simulink model "del3_linjefolging"  (R2024a)
settings: Solver=VariableStepAuto  StartTime=0.0  StopTime=inf  RelTol=1e-3
InitFcn:
  | id_setup()
StartFcn:
  | c_id = evalin('base', "car_id");
  | g_id = evalin('base', "group_id");
  | mqttBasic(c_id,g_id);
libraries: send x3, read x1, init x1
settings Model: Creator=eikel  LastModifiedBy=adriaeik

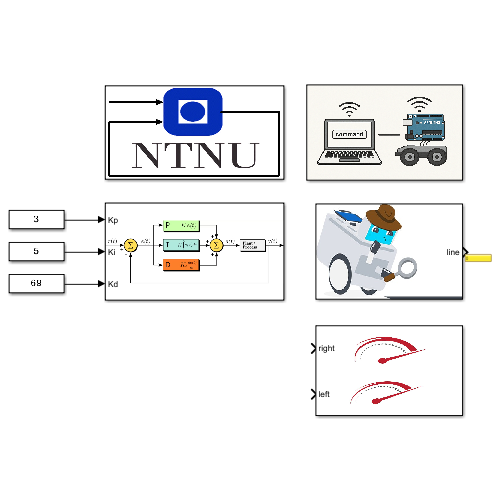
[thumbnail: Simulink's stored preview of the top-level diagram]
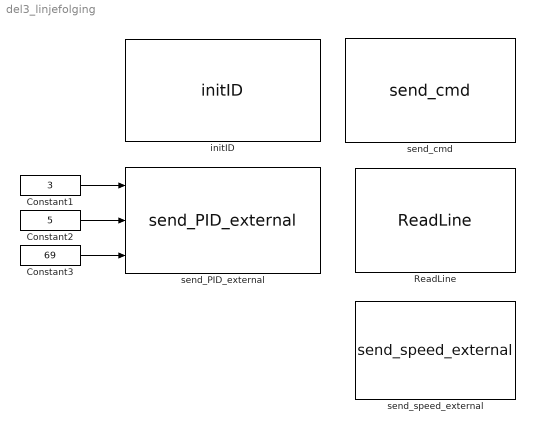
== system del3_linjefolging ==
  Constant1 : Constant  Value=3
  Constant2 : Constant  Value=5
  Constant3 : Constant  Value=69
  ReadLine : read/ReadLine
  initID : init/initID  carID=0  groupID=0
  send_PID_external : send/send_PID_external
  send_cmd : send/send_cmd  cmd=Calibrate
  send_speed_external : send/send_speed_external  SystemSampleTime=-1  VariantActivationTime=update diagram  AllowFlexibleInterface=on  Latency=0  AutoFrameSizeCalculation=off
  wires:
  Constant1/1 -> send_PID_external/1
  Constant2/1 -> send_PID_external/2
  Constant3/1 -> send_PID_external/3
